simulink model "BANG_BANG"  (R2012b)
settings: Solver=ode45  StartTime=0.0  StopTime=20  RelTol=1e-3
settings Model: Creator=Walter  LastModifiedBy=Walter

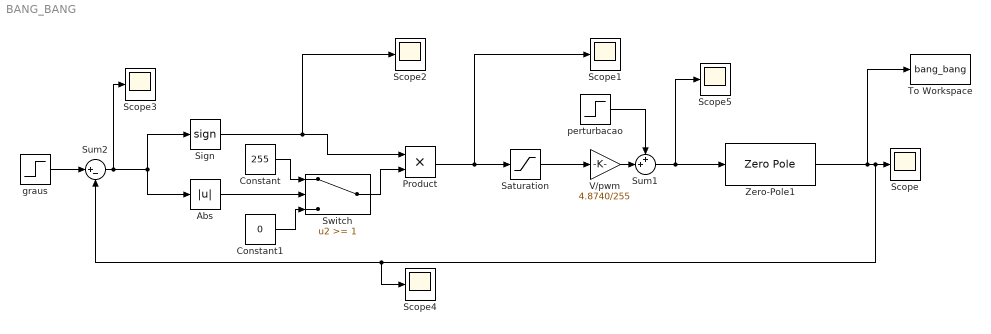
== system BANG_BANG ==
  Abs : Abs
  Constant : Constant  Value=255
  Constant1 : Constant  Value=0
  Product : Product  RndMeth=Zero
  Saturation : Saturate  UpperLimit=255  LowerLimit=-255
  Scope{,1..5} (6 alike) : Scope
      Scope2 settings: SaveName=ScopeData2
      Scope3 settings: SaveName=ScopeData3
      Scope4 settings: SaveName=ScopeData4
      Scope5 settings: SaveName=ScopeData5
  Sign : Signum
  Sum1 : Sum  Inputs=++|
  Sum2 : Sum  Inputs=|+-
  Switch : Switch  Threshold=1
  To Workspace : ToWorkspace  VariableName=bang_bang  SampleTime=-1  SaveFormat=Timeseries
  V/pwm : Gain  Gain=4.8740/255
  Zero-Pole1 : ZeroPole  Zeros=[]  Poles=[0 -15.6250]  Gain=[1725.0719]
  "graus " : Step  Time=0  After=7200
  perturbacao : Step  Time=0  After=0  SampleTime=0
  wires:
  Saturation/1 -> V/pwm/1
  V/pwm/1 -> Sum1/2
  perturbacao/1 -> Sum1/1
  Sum1/1 -> Scope5/1, Zero-Pole1/1
  Zero-Pole1/1 -> To Workspace/1, Scope4/1, Sum2/2, Scope/1
  "graus "/1 -> Sum2/1
  Sign/1 -> Scope2/1, Product/1
  Sum2/1 -> Scope3/1, Abs/1, Sign/1
  Abs/1 -> Switch/2
  Constant1/1 -> Switch/3
  Constant/1 -> Switch/1
  Switch/1 -> Product/2
  Product/1 -> Saturation/1, Scope1/1
